simulink model "Final_Fuzzy_model"  (R2025a)
settings: Solver=ode4  StartTime=0.0  StopTime=1000  FixedStep=0.05  RelTol=1e-3
libraries: fuzblock x1
settings Model: Creator=hero  LastModifiedBy=hero

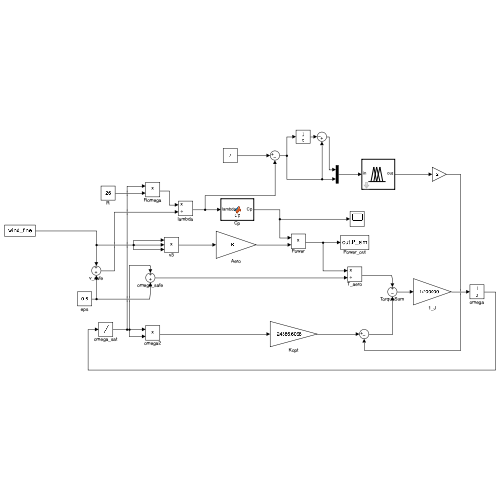
[thumbnail: Simulink's stored preview of the top-level diagram]
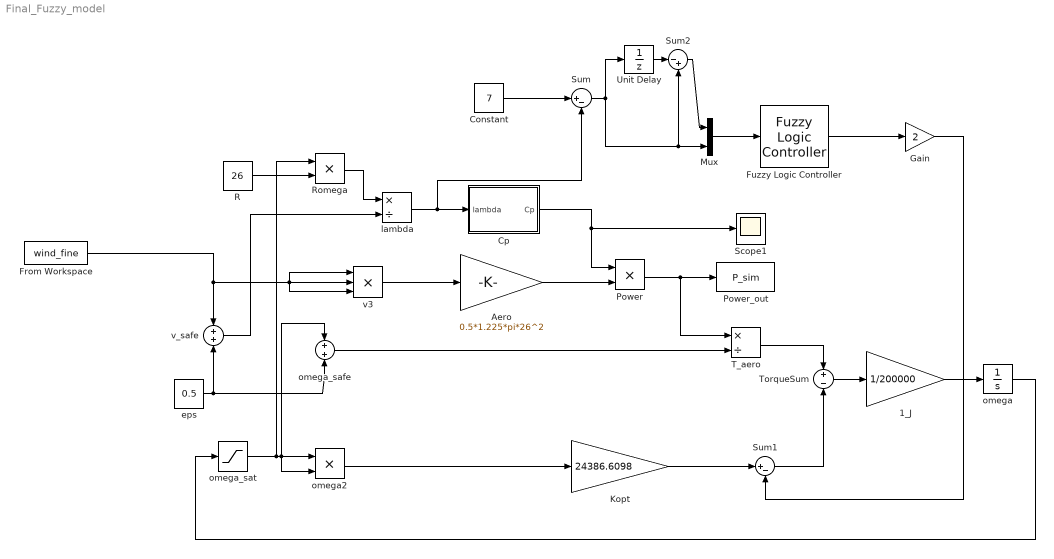
== system Final_Fuzzy_model ==
  1_J : Gain  Gain=1/200000
  Aero : Gain  Gain=0.5*1.225*pi*26^2
  Constant : Constant  Value=7
  Cp : MATLAB Function  TreatAsAtomicUnit=on
  From Workspace : FromWorkspace  VariableName=wind_fine
  Fuzzy Logic Controller : fuzblock/Fuzzy Logic  Controller  FIS=fis  OutputSampleNumber=101  DataType=double  UseLookupTable=off  NumBreakpoints=10  FuzzifiedInputs=off  RuleFiringStrengths=off  RuleOutputs=off  AggregatedOutputs=off  SimulateUsing=Interpreted execution  OutOfRangeInputValueMessage=warning  NoRuleFiredMessage=warning  EmptyOutputFuzzySetMessage=warning
  Gain : Gain  Gain=2
  Kopt : Gain  Gain=24386.6098
  Mux : Mux  Inputs=2
  Power : Product
  Power_out : ToWorkspace  VariableName=P_sim  SampleTime=-1
  R : Constant  Value=26
  Romega : Product
  Scope1 : Scope
      settings: ActiveDisplayYMinimum=-0.00470385215446225  ActiveDisplayYMaximum=0.14095830430867173
  Sum : Sum  Inputs=|+-
  Sum1 : Sum  Inputs=|+-
  Sum2 : Sum  Inputs=|-+
  T_aero : Product  Inputs=*/
  TorqueSum : Sum  Inputs=+-
  Unit Delay : UnitDelay  SampleTime=-1  HasFrameUpgradeWarning=on
  eps : Constant  Value=0.5
  lambda : Product  Inputs=*/
  omega : Integrator  InitialCondition=6
  omega2 : Product
  omega_safe : Sum
  omega_sat : Saturate  UpperLimit=40  LowerLimit=0.5
  v3 : Product  Inputs=3
  v_safe : Sum
  wires:
  omega/1 -> omega_sat/1
  TorqueSum/1 -> 1_J/1
  Power/1 -> T_aero/1, Power_out/1
  Aero/1 -> Power/2
  omega_safe/1 -> T_aero/2
  v3/1 -> Aero/1
  v_safe/1 -> lambda/2
  eps/1 -> omega_safe/2, v_safe/2
  1_J/1 -> omega/1
  omega2/1 -> Kopt/1
  omega_sat/1 -> omega2/1, omega_safe/1, omega2/2, Romega/1
  lambda/1 -> Sum/2, Cp/1(lambda)
  From Workspace/1 -> v3/1, v3/3, v3/2, v_safe/1
  Cp/1(Cp) -> Scope1/1, Power/1
  Romega/1 -> lambda/1
  R/1 -> Romega/2
  Mux/1 -> Fuzzy Logic Controller/1
  Constant/1 -> Sum/1
  Sum/1 -> Unit Delay/1, Sum2/2, Mux/2
  Fuzzy Logic Controller/1 -> Gain/1
  Kopt/1 -> Sum1/1
  Gain/1 -> Sum1/2
  T_aero/1 -> TorqueSum/1
  Sum1/1 -> TorqueSum/2
  Sum2/1 -> Mux/1
  Unit Delay/1 -> Sum2/1

== matlab function Final_Fuzzy_model/Cp ==
  data: lambda input; Cp output
function Cp = Cp(lambda)
lambda = max(lambda,0.1);
lambda_i = 1./(1./(lambda+0.08) - 0.035./(lambda.^3 + 1));
Cp = 0.22*((116./lambda_i)-5).*exp(-12.5./lambda_i);
Cp = max(0,min(0.59,Cp));
end
